simulink model "model"  (R2020b)
settings: Solver=VariableStepAuto  StartTime=0.0  StopTime=inf  RelTol=1e-3
settings Model: Creator=Pavan  LastModifiedBy=Pavan

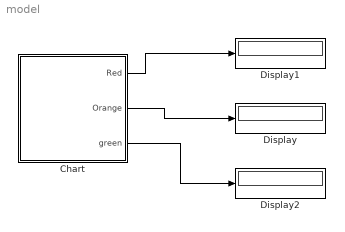
== system model ==
  Chart : Stateflow chart  TreatAsAtomicUnit=on
  Display : Display
  Display1 : Display
  Display2 : Display
  wires:
  Chart/2(Orange) -> Display/1
  Chart/1(Red) -> Display1/1
  Chart/3(green) -> Display2/1

== stateflow chart model/Chart ==
  state Go
    en: Red =0;
    Orange =0;
    green =1;
  state SlowDown
    en:Red =0;
    Orange =1;
    green =0;
  state Stop
    en: Red =1;
    Orange =0;
    green =0;
  (default) -> Go
  Go -> SlowDown : after(100000,sec)
  SlowDown -> Stop : after(50000,sec)
  Stop -> Go : after(100000,sec)
  data: Red output; Orange output; green output
